simulink model "Session_LAB"  (R2021a)
settings: Solver=VariableStepAuto  StartTime=0.0  StopTime=20.0  MaxStep=1e-3  RelTol=1e-3
settings Model: Creator=MAC  LastModifiedBy=MAC

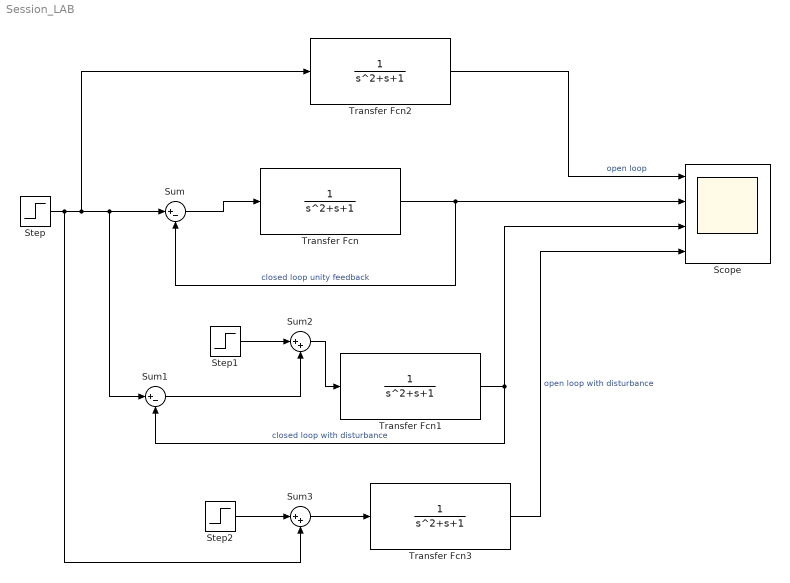
== system Session_LAB ==
  Scope : Scope  NumInputPorts=4
  Step : Step  SampleTime=0
  Step1 : Step  SampleTime=0
  Step2 : Step  SampleTime=0
  Sum : Sum  Inputs=|+-
  Sum1 : Sum  Inputs=|+-
  Sum2 : Sum  Inputs=|++
  Sum3 : Sum  Inputs=|++
  Transfer Fcn{,1..3} (4 alike) : TransferFcn  Denominator=[1 1 1]
  wires:
  Transfer Fcn/1 -> Scope/2, Sum/2  "closed loop unity feedback"
  Sum/1 -> Transfer Fcn/1
  Transfer Fcn2/1 -> Scope/1  "open loop"
  Transfer Fcn1/1 -> Scope/3, Sum1/2  "closed loop with disturbance"
  Step/1 -> Sum3/2, Transfer Fcn2/1, Sum1/1, Sum/1
  Step1/1 -> Sum2/1
  Sum1/1 -> Sum2/2
  Sum2/1 -> Transfer Fcn1/1
  Step2/1 -> Sum3/1
  Sum3/1 -> Transfer Fcn3/1
  Transfer Fcn3/1 -> Scope/4  "open loop with disturbance"
